simulink model "admire_sim_NDI"  (Simulink 9.1)
settings: Solver=ode4  StartTime=0.0  StopTime=500  FixedStep=dt  RelTol=1e-3  AbsTol=1e-6
InitFcn:
  | INIT_NDI
StartFcn:
  | tic
StopFcn:
  | toctime=toc;
  | fprintf('Actual Time = %g\nSim Time = %g\n',toctime,tout(end))
  | % Make plots
  | %admire_sim_plot
  | figure
  | plot3(yout(:,11),yout(:,10),-yout(:,12),'*-');grid
  | xlabel('East (m)');ylabel('North (m)');zlabel('Alt (m)')
  | view([0 0 1])
  | hold on
  | plot3(Ywpt,Xwpt,0*Xwpt,'r^-','MarkerSize',10)
  | axis equal
  | hold off
values from neighbouring files (symbols this model uses):
  a1 = (180*d2r)/(80^3)    (= 6.13592315154e-06)    [INIT_NDI.m]
  a2 = (24*d2r)/(80^3)    (= 8.18123086872e-07)    [INIT_NDI.m]
  Altcmd_t = [ 0    1   100 200  300  425  450  550  600  700  800  880  980]    [INIT_NDI.m]
  Altcmd_v = [20  20   20   1500 1500 1500 1500 3000 3000 4000 4000 6000 6000]    [INIT_NDI.m]
  bref = 10    [INIT_NDI.m]
  C1 = ((Iy-Iz)*Iz-Ixz^2)/GG    (= -0.958151081688)    [INIT_NDI.m]
  C2 = (Ix-Iy+Iz)*Ixz/GG    (= 0.0484690861804)    [INIT_NDI.m]
  C3 = Iz/GG    (= 4.77597824802e-05)    [INIT_NDI.m]
  C4 = Ixz/GG    (= 1.18217283367e-06)    [INIT_NDI.m]
  C5 = (Iz-Ix)/Iy    (= 0.987654320988)    [INIT_NDI.m]
  C6 = Ixz/Iy    (= 0.0308641975309)    [INIT_NDI.m]
  C7 = 1/Iy    (= 1.23456790123e-05)    [INIT_NDI.m]
  C8 = (Ix*(Ix-Iy)+Ixz^2)/GG    (= -0.592859676085)    [INIT_NDI.m]
  C9 = Ix/GG    (= 9.93025180281e-06)    [INIT_NDI.m]
  CAmethod = 6    [INIT_NDI.m]
  Canard_max = [25 25 25 15 15 15 15 15]*d2r    [INIT_NDI.m]
  Canard_min = [-55 -55 -25 -15 -15 -15 -15 -15]*d2r    [INIT_NDI.m]
  CB = CCV*Bbare    [INIT_NDI.m]
  CC = [C3 0 C4;0 C7 0;C4 0 C9]    [INIT_NDI.m]
  CCV = [CCV zeros(3,22)]    [INIT_NDI.m]
  cref = 5.2    [INIT_NDI.m]
  d2r = pi/180    (= 0.0174532925199)    [INIT_NDI.m]
  dt = 0.01    [INIT_NDI.m]
  DTY_max = 0.002    [INIT_NDI.m]
  DTY_min = -0.002    [INIT_NDI.m]
  DTZ_max = 0.002    [INIT_NDI.m]
  DTZ_min = -0.002    [INIT_NDI.m]
  du = [eye(7,7)*d2r eye(7,7)*(-d2r);zeros(20,14)]    [INIT_NDI.m]
  Elevon_max = [30 30 25 25 25 25 25 25]*d2r    [INIT_NDI.m]
  Elevon_min = [-30 -30 -30 -30 -30 -30 -30 -30]*d2r    [INIT_NDI.m]
  G = [ 0 1 0 ... (first row only)    [INIT_NDI.m]
  kcb = 2.5    [INIT_NDI.m]
  kfb = -0.4    [INIT_NDI.m]
  kib = 0.2    [INIT_NDI.m]
  kpb = 0.8    [INIT_NDI.m]
  LEF_max = [30 30 30 20 20 15 10 10]*d2r    [INIT_NDI.m]
  LEF_min = [-10 -10 -10 -10 -10 -10 -10 -10]*d2r    [INIT_NDI.m]
  LG_max = 1    [INIT_NDI.m]
  LG_min = 0    [INIT_NDI.m]
  LPmethod = 5    [INIT_NDI.m]    (also in LPwrap.m = 0)
  M_vec = [0 0.5 0.8 0.9 0.95 1.4 1.5 2.5]    [INIT_NDI.m]
  mass = 9100    [INIT_NDI.m]
  NumU = 16    [INIT_NDI.m]
  nwpt = 5    [INIT_NDI.m]
  PD_max = 10    [INIT_NDI.m]
  PD_min = -10    [INIT_NDI.m]
  PHIcmd_t = [0 1 1+dt 30 30+dt 60 60+dt 90 90+dt 120 120+dt 150 150+dt 180 180+dt 210 210+dt 240 240+dt 270 270+dt 300 300+dt 330 330+dt]    [INIT_NDI.m]
  PHIcmd_v = [0 0 15   15 -15   -15 0    0   30   30  -30    -30 0      0   45     45   0     0    -45   -45   0     0   -60   -60 0]    [INIT_NDI.m]
  Pmode = 3    [INIT_NDI.m]
  r2d = 180/pi    (= 57.2957795131)    [INIT_NDI.m]
  Rmode = 3    [INIT_NDI.m]
  Rudder_max = [30 30 25 20 15 15 15 10]*d2r    [INIT_NDI.m]
  Rudder_min = [-30 -30 -25 -20 -15 -15 -15 -10]*d2r    [INIT_NDI.m]
  Sref = 45    [INIT_NDI.m]
  TSS_max = 1    [INIT_NDI.m]
  TSS_min = 0    [INIT_NDI.m]
  UD_max = 10    [INIT_NDI.m]
  UD_min = -10    [INIT_NDI.m]
  Upref = [0 0 0 0 0 0 0 0 0 0 0 0 0 0 0 0]'    [INIT_NDI.m]
  Upref_split = [[0 0 30 -30 -30 30 0]*d2r*.4 0 0 0 0 0 0 0 0 0]'    [INIT_NDI.m]
  Urlim = [50*d2r ... (first row only)    [INIT_NDI.m]
  UseRL = 0    [INIT_NDI.m]
  Vcmd_t = [  0    1   100  200  300  425  450  550  600  700  800  880  980]    [INIT_NDI.m]
  Vcmd_v = Mcmd_v.*a    [INIT_NDI.m]
  VD_max = 10    [INIT_NDI.m]
  VD_min = -10    [INIT_NDI.m]
  WD_max = 10    [INIT_NDI.m]
  WD_min = -10    [INIT_NDI.m]
  Wp = W'*W    [INIT_NDI.m]
  Wpts = [0 1 2 3 4]    [INIT_NDI.m]
  x0 = [ max(eyp,zeros(n,1));max(-eyp,zeros(n,1));zeros(2*m,1)]    [LPwrap.m]
  Xwpt = [0 4000 4000 0 0]*8    [INIT_NDI.m]
  Ywpt = [0 0 4000 4000 0]*8    [INIT_NDI.m]
undefined symbols (not defined in the file or in its folder): Abare, Bbare, CGIwrap, dalpha_err, dalt_err, DAwrap, dbeta_err, ddc_bw, ddc_rate, ddei_bw, ddei_rate, ddey_bw, ddey_rate, ddle_bw, ddle_rate, ddr_bw, ddr_rate, DiscIntNeverNeededParam, dVt_err, LPwrap, rlimit_c, rlimit_ie, rlimit_le, rlimit_oe, rlimit_r, u0fcs, u0new, VJAwrap, x0bare, y0bare
libraries: simulink_extras x19, simulink x12
(part 3 of 4)

== system admire_sim_NDI/NDI_CLAW/DynamicInversionControl/REG/PitchReg/QCMD_1 ==
  CMD : Inport
  INPUT : Inport  Port=2
  Action Port : ActionPort  ActionType=then
  1-D Lookup Table : Lookup_n-D  NumberOfTableDimensions=1  BreakpointsForDimension1=[0.4 0.6 0.8]  Table=[30 40 50]  ExtrapMethod=Clip  UseLastTableValue=on  RndMeth=Simplest  InputSameDT=on
  Bus Selector1 : BusSelector  OutputSignals=PSTICK
  Bus Selector2 : BusSelector  OutputSignals=Mach
  Bus Selector4 : BusSelector  OutputSignals=Qb_rps
  Bus Selector5 : BusSelector  OutputSignals=Reset
  Discrete-Time Integrator1 : DiscreteIntegrator  IntegratorMethod=Integration: Trapezoidal  ExternalReset=level  SampleTime=dt  ICPrevOutput=DiscIntNeverNeededParam  ICPrevScaledInput=DiscIntNeverNeededParam
  Gain2 : Gain  Gain=6
  Gain3 : Gain  Gain=5
  Gain4 : Gain  Gain=d2r
  Gain5 : Gain  Gain=-1
  Gain6 : Gain  Gain=80
  Product : Product  RndMeth=Zero
  QCMD_Gradient : Lookup_n-D  NumberOfTableDimensions=1  BreakpointsForDimension1=[-80:80]  Table=a2*([-80:80].^3)  ExtrapMethod=Clip  UseLastTableValue=on  RndMeth=Simplest  InputSameDT=on
  Sum : Sum  Inputs=+++
  Sum2 : Sum  Inputs=|+-
  MCVdt : Outport
  wires:
  CMD/1 -> Bus Selector1/1, Bus Selector5/1
  QCMD_Gradient/1 -> Sum2/1, Gain5/1  "Qcmd"
  Sum2/1 -> Gain2/1, Gain3/1
  Sum/1 -> MCVdt/1  "QDT_des"
  INPUT/1 -> Bus Selector2/1, Bus Selector4/1
  Bus Selector2/1 -> 1-D Lookup Table/1  "<Mach>"
  1-D Lookup Table/1 -> Product/2
  Bus Selector1/1 -> Gain6/1, Product/1  "<PSTICK>"
  Product/1 -> Gain4/1
  Bus Selector5/1 -> Discrete-Time Integrator1/2  "<Reset>"
  Discrete-Time Integrator1/1 -> Sum/2
  Gain2/1 -> Sum/3
  Gain3/1 -> Discrete-Time Integrator1/1
  Gain5/1 -> Sum/1
  Gain6/1 -> QCMD_Gradient/1
  Bus Selector4/1 -> Sum2/2  "<Qb_rps>"

== system admire_sim_NDI/NDI_CLAW/DynamicInversionControl/REG/RollReg/PHIcmd_2 ==
  CMD : Inport
  INPUT : Inport  Port=2
  Action Port : ActionPort  ActionType=elseif
  Bus Selector2 : BusSelector  OutputSignals=PHIcmd_rad
  Bus Selector3 : BusSelector  OutputSignals=PHI_rad
  Bus Selector5 : BusSelector  OutputSignals=Reset
  Constant : Constant  Value=100*d2r
  Discrete-Time Integrator1 : DiscreteIntegrator  IntegratorMethod=Integration: Trapezoidal  ExternalReset=level  SampleTime=dt  ICPrevOutput=DiscIntNeverNeededParam  ICPrevScaledInput=DiscIntNeverNeededParam
  Gain1 : Gain  Gain=5
  Gain3 : Gain  Gain=1.6
  Gain7 : Gain  Gain=-0.8
  Gain8 : Gain  Gain=.8
  Get_LCV : Subsystem
  Sum1 : Sum  Inputs=|+-
  Sum2 : Sum  Inputs=|+-
  Sum3 : Sum  Inputs=++|
  Sum4 : Sum  Inputs=++|
  VariableLimiter : Subsystem
  LCVdt : Outport
  wires:
  CMD/1 -> Bus Selector5/1, Bus Selector2/1
  Sum1/1 -> Gain8/1, Gain3/1
  Bus Selector3/1 -> Sum1/2  "<PHI_rad>"
  Sum2/1 -> Gain1/1
  Gain1/1 -> LCVdt/1  "Pdt_des"
  VariableLimiter/1(Out) -> Sum2/1  "Pcmd_lim"
  Constant/1 -> VariableLimiter/2(Limit)
  Get_LCV/1(LCV) -> Sum2/2
  INPUT/1 -> Get_LCV/1(Input), Bus Selector3/1
  Bus Selector5/1 -> Discrete-Time Integrator1/2  "<Reset>"
  Gain3/1 -> Sum4/2  "Pcmd"
  Sum4/1 -> VariableLimiter/1(Input)
  Gain8/1 -> Discrete-Time Integrator1/1
  Discrete-Time Integrator1/1 -> Sum3/2
  Sum3/1 -> Sum4/1
  Gain7/1 -> Sum3/1
  Bus Selector2/1 -> Sum1/1, Gain7/1  "<PHIcmd_rad>"

== system admire_sim_NDI/NDI_CLAW/DynamicInversionControl/REG/RollReg/Pcmd_1 ==
  CMD : Inport
  INPUT : Inport  Port=2
  Action Port : ActionPort  ActionType=then
  1-D Lookup Table : Lookup_n-D  NumberOfTableDimensions=1  BreakpointsForDimension1=[0.4 0.6 0.8]  Table=[50 100 180]  ExtrapMethod=Clip  UseLastTableValue=on  RndMeth=Simplest  InputSameDT=on
  Bus Selector2 : BusSelector  OutputSignals=RSTICK
  Bus Selector3 : BusSelector  OutputSignals=Mach
  Constant : Constant  Value=100*d2r
  Gain1 : Gain  Gain=2
  Gain2 : Gain  Gain=d2r
  Gain3 : Gain  Gain=80
  Get_LCV : Subsystem
  PCMD_Gradient : Lookup_n-D  NumberOfTableDimensions=1  BreakpointsForDimension1=[-80:80]  Table=a1*([-80:80].^3)  ExtrapMethod=Clip  UseLastTableValue=on  RndMeth=Simplest  InputSameDT=on
  Product : Product  RndMeth=Zero
  Sum2 : Sum  Inputs=|+-
  Terminator : Terminator
  VariableLimiter : Subsystem
  LCVdt : Outport
  wires:
  Get_LCV/1(LCV) -> Sum2/2
  PCMD_Gradient/1 -> Sum2/1  "Pcmd_lim"
  Gain1/1 -> LCVdt/1  "Pdt_des"
  Sum2/1 -> Gain1/1
  Product/1 -> Gain2/1  "Pcmd_dps"
  Bus Selector2/1 -> Product/1, Gain3/1  "<RSTICK>"
  CMD/1 -> Bus Selector2/1
  Gain2/1 -> VariableLimiter/1(Input)  "Pcmd_rps"
  INPUT/1 -> Get_LCV/1(Input), Bus Selector3/1
  Bus Selector3/1 -> 1-D Lookup Table/1  "<Mach>"
  1-D Lookup Table/1 -> Product/2
  Constant/1 -> VariableLimiter/2(Limit)
  Gain3/1 -> PCMD_Gradient/1
  VariableLimiter/1(Out) -> Terminator/1  "Pcmd_lim"

== system admire_sim_NDI/NDI_CLAW/DynamicInversionControl/REG/RollReg/XTKcmd_3 ==
  CMD : Inport
  INPUT : Inport  Port=2
  Action Port : ActionPort  ActionType=else
  Bus Selector3 : BusSelector  OutputSignals=PHI_rad
  Constant : Constant  Value=100*d2r
  Gain1 : Gain  Gain=3
  Gain3 : Gain  Gain=.75
  GetPHIcmd : Subsystem
  Get_LCV : Subsystem
  Sum1 : Sum  Inputs=|+-
  Sum2 : Sum  Inputs=|+-
  VariableLimiter : Subsystem
  LCVdt : Outport
  wires:
  Get_LCV/1(LCV) -> Sum2/2
  Constant/1 -> VariableLimiter/2(Limit)
  VariableLimiter/1(Out) -> Sum2/1  "Pcmd_lim"
  Gain1/1 -> LCVdt/1  "Pdt_des"
  Sum2/1 -> Gain1/1
  Bus Selector3/1 -> Sum1/2  "<PHI_rad>"
  Gain3/1 -> VariableLimiter/1(Input)  "Pcmd"
  Sum1/1 -> Gain3/1
  GetPHIcmd/1(PHIcmd) -> Sum1/1
  CMD/1 -> GetPHIcmd/1(CMD)
  INPUT/1 -> Get_LCV/1(Input), Bus Selector3/1, GetPHIcmd/2(INPUT)

== system admire_sim_NDI/NDI_CLAW/DynamicInversionControl/REG/YawReg/Get_NCV ==
  Input : Inport
  Bus Selector4 : BusSelector  OutputSignals=Rb_rps,ALPHA_rad,Pb_rps,VT_mps,PHI_rad,THETA_rad
  Constant : Constant
  Gain : Gain  Gain=9.81
  MinMax : MinMax  Function=max  Inputs=2
  Product : Product  RndMeth=Zero
  Product1 : Product  RndMeth=Zero
  Product2 : Product  Inputs=/**  RndMeth=Zero
  Sum4 : Sum  Inputs=|+-
  Sum5 : Sum  Inputs=|+-
  Trigonometric Function : Trigonometry
  Trigonometric Function1 : Trigonometry  Operator=cos
  Trigonometric Function2 : Trigonometry
  Trigonometric Function3 : Trigonometry  Operator=cos
  NCV : Outport
  wires:
  Bus Selector4/2 -> Trigonometric Function/1, Trigonometric Function1/1  "<ALPHA_rad>"
  Trigonometric Function1/1 -> Product/2
  Trigonometric Function/1 -> Product1/1
  Product/1 -> Sum4/1
  Product1/1 -> Sum4/2
  Constant/1 -> MinMax/2
  Bus Selector4/4 -> MinMax/1  "<VT_mps>"
  Bus Selector4/5 -> Trigonometric Function2/1  "<PHI_rad>"
  Bus Selector4/6 -> Trigonometric Function3/1  "<THETA_rad>"
  MinMax/1 -> Product2/1
  Trigonometric Function2/1 -> Product2/2
  Trigonometric Function3/1 -> Product2/3
  Product2/1 -> Gain/1
  Sum4/1 -> Sum5/1
  Gain/1 -> Sum5/2
  Input/1 -> Bus Selector4/1
  Bus Selector4/1 -> Product/1  "<Rb_rps>"
  Bus Selector4/3 -> Product1/2  "<Pb_rps>"
  Sum5/1 -> NCV/1

== system admire_sim_NDI/NDI_CLAW/MissionManager/WaypointNavigation/ChangeWptNumber/GetTurnDist ==
  INPUT : Inport
  WNz : Inport  Port=2
  Bus Selector2 : BusSelector  OutputSignals=VT_mps  OutputAsBus=on
  GetHalfAngle : Subsystem
  GetPHILimit : Subsystem
  GetRadius : Subsystem
  Product : Product  RndMeth=Zero
  Product4 : Product  Inputs=**/  RndMeth=Zero
  Trigonometric Function1 : Trigonometry  Operator=cos
  Trigonometric Function2 : Trigonometry
  V2 : Outport
  TurnDist_m : Outport  Port=2
  PHImax_rad : Outport  Port=3
  wires:
  Bus Selector2/1 -> Product/1, Product/2
  Product/1 -> V2/1, GetRadius/1(V2), GetPHILimit/1(V2)
  GetPHILimit/1(PHImax_rad) -> GetRadius/2(PHImax_rad), PHImax_rad/1
  INPUT/1 -> Bus Selector2/1
  WNz/1 -> GetHalfAngle/1(WNz)
  GetHalfAngle/1(Out1) -> Trigonometric Function1/1, Trigonometric Function2/1
  GetRadius/1(R_m) -> Product4/1
  Trigonometric Function1/1 -> Product4/2
  Trigonometric Function2/1 -> Product4/3
  Product4/1 -> TurnDist_m/1  "TurnDist_m"

== system admire_sim_NDI/NDI_CLAW/DynamicInversionControl/AERO_OBM/NonLinearOBM/Get_B_Aero/Dimensions ==
  note: Generate a matrix which will multiply
      | the moment coefficients to turn them
      | into properly dimensioned moments
  In1 : Inport
  Gain1 : Gain  Gain=-1
  Gain2 : Gain  Gain=0.5
  Gain3 : Gain  Gain=bref
  Gain4 : Gain  Gain=bref
  Gain5 : Gain  Gain=cref
  Gain6 : Gain  Gain=Sref
  Gain7 : Gain  Gain=[1 1 1]  Multiplication=Matrix(u*K)
  Gain8 : Gain  Gain=eye(3,3)
  GetDensity : Subsystem
  Mux1 : Mux  Inputs=3
  Product : Product  RndMeth=Zero
  Product1 : Product  RndMeth=Zero
  Selector4 : Selector  InputPortWidth=27  IndexOptions=Index vector (dialog)  Indices=[19]  OutputSizes=1
  Selector5 : Selector  InputPortWidth=27  IndexOptions=Index vector (dialog)  Indices=[13]  OutputSizes=1
  Out1 : Outport
  wires:
  Selector4/1 -> Gain1/1
  Gain1/1 -> GetDensity/1(Alt_m)  "Alt_m"
  Selector5/1 -> Product/1, Product/2
  Product/1 -> Gain2/1
  GetDensity/1(rho_kpm3) -> Product1/1
  Gain2/1 -> Product1/2  "V*V*0.5"
  Gain5/1 -> Mux1/2
  Gain3/1 -> Mux1/1
  Gain4/1 -> Mux1/3
  Product1/1 -> Gain3/1, Gain5/1, Gain4/1  "dynamic pressure"
  Mux1/1 -> Gain6/1
  In1/1 -> Selector4/1, Selector5/1
  Gain6/1 -> Gain7/1
  Gain7/1 -> Gain8/1
  Gain8/1 -> Out1/1

== system admire_sim_NDI/NDI_CLAW/DynamicInversionControl/AERO_OBM/NonLinearOBM/Get_B_Aero/Get_CVdt ==
  Dim : Inport
  Sensors : Inport  Port=2
  uz : Inport  Port=3
  DueToEffectors : Subsystem
  Sum : Sum  Inputs=|+-
  TotalAccels : Subsystem
  CVdt : Outport
  wires:
  DueToEffectors/1(Out1) -> Sum/2  "B*u-B*u_nom"
  Sum/1 -> CVdt/1
  uz/1 -> DueToEffectors/3(uz)
  Dim/1 -> DueToEffectors/2(Dim), TotalAccels/1(Dim)
  Sensors/1 -> DueToEffectors/1(Sensors), TotalAccels/2(Sensors)
  TotalAccels/1(CVdt) -> Sum/1  "f(x,u)"

== system admire_sim_NDI/NDI_CLAW/DynamicInversionControl/AERO_OBM/NonLinearOBM/Get_B_Aero/OneColPerFrame ==
  In1 : Inport
  In2 : Inport  Port=2
  Bz : Inport  Port=3
  Assignment : Assignment  NumberOfDimensions=2  IndexOptions=Index vector (dialog),Index vector (port)  Indices=[1 2 3],1  OutputSizes=1,1
  Merge : Merge  Inputs=7
  Signal Specification : SignalSpecification  Dimensions=[3 1]
  Switch Case : SwitchCase  CaseConditions={7,6,5,4,3,2,1}  ShowDefaultCase=off  SampleTime=0
  u1 : Subsystem
  u2 : Subsystem
  u3 : Subsystem
  u4 : Subsystem
  u5 : Subsystem
  u6 : Subsystem
  u7 : Subsystem
  Out1 : Outport
  wires:
  In1/1 -> u1/1(In1), u2/1(In1), u3/1(In1), u4/1(In1), u5/1(In1), u7/1(In1), u6/1(In1)
  u1/1(Out1) -> Merge/1
  u2/1(Out1) -> Merge/2
  u3/1(Out1) -> Merge/3
  u4/1(Out1) -> Merge/4
  u5/1(Out1) -> Merge/5
  u6/1(Out1) -> Merge/6
  u7/1(Out1) -> Merge/7
  Switch Case/1 -> u7/Action
  Switch Case/2 -> u6/Action
  Switch Case/3 -> u5/Action
  Switch Case/4 -> u4/Action
  Switch Case/5 -> u3/Action
  Switch Case/6 -> u2/Action
  Switch Case/7 -> u1/Action
  In2/1 -> Assignment/3, Switch Case/1
  Bz/1 -> Assignment/1
  Assignment/1 -> Out1/1
  Merge/1 -> Signal Specification/1
  Signal Specification/1 -> Assignment/2

== system admire_sim_NDI/NDI_CLAW/DynamicInversionControl/ControlAllocation/GetU/MakeSquare_0/Subsystem ==
  In1 : Inport
  Bus Selector1 : BusSelector  OutputSignals=CB
  Bus Selector3 : BusSelector  OutputSignals=INDX
  Constant : Constant  Value=G
  Math Function2 : Math  Operator=transpose  SaturateOnIntegerOverflow=on
  Matrix Concatenate : Concatenate  NumInputs=3  Mode=Multidimensional array
  Product : Product
  Product1 : Product  Multiplication=Matrix(*)
  Signal Specification1 : SignalSpecification  Dimensions=[1 NumU]
  Gmod : Outport
  CBGmod : Outport  Port=2
  wires:
  Math Function2/1 -> Product/2
  Bus Selector3/1 -> Signal Specification1/1  "<INDX>"
  Signal Specification1/1 -> Matrix Concatenate/1, Matrix Concatenate/2, Matrix Concatenate/3
  Product/1 -> Product1/2, Gmod/1
  Matrix Concatenate/1 -> Math Function2/1
  Constant/1 -> Product/1
  Bus Selector1/1 -> Product1/1  "<CB>"
  In1/1 -> Bus Selector1/1, Bus Selector3/1
  Product1/1 -> CBGmod/1

== system admire_sim_NDI/NDI_CLAW/DynamicInversionControl/ControlAllocation/GetU/WeightedPseudo Clipped_1/GetP ==
  CB : Inport
  WpT : Inport  Port=2
  CBT : Inport  Port=3
  Product : Product  Inputs=/*  Multiplication=Matrix(*)  RndMeth=Zero
  Product1 : Product  Inputs=**  Multiplication=Matrix(*)  RndMeth=Zero
  Product2 : Product  Inputs=*/  Multiplication=Matrix(*)  RndMeth=Zero
  P : Outport
  wires:
  CBT/1 -> Product/2
  Product2/1 -> P/1  "P"
  WpT/1 -> Product/1
  CB/1 -> Product1/1
  Product1/1 -> Product2/2
  Product/1 -> Product2/1, Product1/2

== system admire_sim_NDI/NDI_CLAW/DynamicInversionControl/ControlAllocation/GetU/WeightedPseudo Clipped_1/SelectActive ==
  In1 : Inport
  Bus Selector2 : BusSelector  OutputSignals=CB
  Bus Selector3 : BusSelector  OutputSignals=INDX
  Matrix Concatenate : Concatenate  NumInputs=3  Mode=Multidimensional array
  Product : Product
  Signal Specification1 : SignalSpecification  Dimensions=[1 NumU]
  Out1 : Outport
  wires:
  Matrix Concatenate/1 -> Product/1
  Product/1 -> Out1/1
  Bus Selector3/1 -> Signal Specification1/1  "<INDX>"
  Bus Selector2/1 -> Product/2  "<CB>"
  In1/1 -> Bus Selector3/1, Bus Selector2/1
  Signal Specification1/1 -> Matrix Concatenate/3, Matrix Concatenate/2, Matrix Concatenate/1

== system admire_sim_NDI/NDI_CLAW/DynamicInversionControl/ControlAllocation/GetU/WeightedPseudo Scaled_2/Blocks ==
  CB : Inport
  CVdt_des : Inport  Port=2
  Umin : Inport  Port=3
  Umax : Inport  Port=4
  Wp : Inport  Port=5
  CheckSaturation : Subsystem
  GetP : Subsystem
  If : If  IfExpression=u1 < 1
  Math Function : Math  Operator=transpose  SaturateOnIntegerOverflow=on
  Math Function1 : Math  Operator=transpose  SaturateOnIntegerOverflow=on
  Merge : Merge
  None_Saturated : Subsystem  TreatAsAtomicUnit=on
  Product3 : Product  Inputs=**  Multiplication=Matrix(*)  RndMeth=Zero
  Some_Saturated : Subsystem  TreatAsAtomicUnit=on
  Out1 : Outport
  wires:
  Merge/1 -> Out1/1
  Umin/1 -> Some_Saturated/2(umin), CheckSaturation/2(Umin)
  Umax/1 -> Some_Saturated/1(umax), CheckSaturation/3(Umax)
  None_Saturated/1(Out1) -> Merge/2
  Some_Saturated/1(Out1) -> Merge/1
  If/1 -> None_Saturated/Action
  If/2 -> Some_Saturated/Action
  CheckSaturation/1(Out1) -> If/1
  Product3/1 -> CheckSaturation/1(In1), Some_Saturated/3(u), None_Saturated/1(In1)  "u"
  CVdt_des/1 -> Product3/2
  GetP/1(P) -> Product3/1
  Math Function1/1 -> GetP/3(CBT)
  Math Function/1 -> GetP/2(WpT)
  Wp/1 -> Math Function/1
  CB/1 -> GetP/1(CB), Math Function1/1

== system admire_sim_NDI/NDI_CLAW/DynamicInversionControl/ControlAllocation/GetU/WeightedPseudo Scaled_2/SelectActive ==
  In1 : Inport
  Bus Selector2 : BusSelector  OutputSignals=CB
  Bus Selector3 : BusSelector  OutputSignals=INDX
  Matrix Concatenate : Concatenate  NumInputs=3  Mode=Multidimensional array
  Product : Product
  Signal Specification1 : SignalSpecification  Dimensions=[1 NumU]
  Out1 : Outport
  wires:
  Matrix Concatenate/1 -> Product/1
  Product/1 -> Out1/1
  Bus Selector3/1 -> Signal Specification1/1  "<INDX>"
  Bus Selector2/1 -> Product/2  "<CB>"
  In1/1 -> Bus Selector3/1, Bus Selector2/1
  Signal Specification1/1 -> Matrix Concatenate/3, Matrix Concatenate/2, Matrix Concatenate/1

== system admire_sim_NDI/NDI_CLAW/DynamicInversionControl/ControlAllocation/PostProcess/DriveToPreferred/Get_UPerp ==
  In1 : Inport
  In2 : Inport  Port=2
  Bus Selector3 : BusSelector  OutputSignals=CB,INDX
  MATLAB Fcn : MATLABFcn  MATLABFcn=getUperp  Output1D=off
  Math Function1 : Math  Operator=transpose  SaturateOnIntegerOverflow=on
  Math Function3 : Math  Operator=transpose  SaturateOnIntegerOverflow=on
  Matrix Concatenate : Concatenate  NumInputs=3  Mode=Multidimensional array
  Signal Specification1 : SignalSpecification  Dimensions=[NumU 1]
  Signal Specification3 : SignalSpecification  Dimensions=[NumU 1]
  Out1 : Outport
  wires:
  Signal Specification3/1 -> Math Function3/1
  Matrix Concatenate/1 -> MATLAB Fcn/1
  In1/1 -> Bus Selector3/1
  Bus Selector3/2 -> Signal Specification3/1  "<INDX>"
  MATLAB Fcn/1 -> Out1/1
  Bus Selector3/1 -> Matrix Concatenate/1  "<CB>"
  In2/1 -> Signal Specification1/1
  Signal Specification1/1 -> Math Function1/1
  Math Function1/1 -> Matrix Concatenate/2
  Math Function3/1 -> Matrix Concatenate/3

== system admire_sim_NDI/NDI_CLAW/DynamicInversionControl/ControlAllocation/PostProcess/DriveToPreferred/LimitScale ==
  note: Deal with the situation where K_opt*u_perp is already the optimal solution, at this time the gain is greater than 1
  Vector : Inport
  MinValues : Inport  Port=2
  MaxValues : Inport  Port=3
  PrePro : Inport  Port=4
  Abs1 : Abs
  "Calculate the gain factor to the lower limit " : Subsystem
  "Calculate the gain factor to the upper limit " : Subsystem
  Compare To Zero : simulink/Logic and Bit Operations/Compare To Zero  relop=<  OutDataTypeStr=uint8
  Compare To Zero1 : simulink/Logic and Bit Operations/Compare To Zero  relop=>=  OutDataTypeStr=uint8
  Constant : Constant
  Data Type Conversion1 : DataTypeConversion  OutDataTypeStr=double
  Data Type Conversion2 : DataTypeConversion  OutDataTypeStr=double
  DivideByZeroProtection : Subsystem
  MinMax : MinMax
  Mux : Mux  Inputs=2
  Product : Product  RndMeth=Zero
  Product1 : Product  RndMeth=Zero
  Sign : Signum
  Sum : Sum  Inputs=|++
  Scale : Outport
  wires:
  Abs1/1 -> MinMax/1
  MinMax/1 -> Scale/1
  Vector/1 -> DivideByZeroProtection/1(In1)
  DivideByZeroProtection/1(Out1) -> "Calculate the gain factor to the lower limit "/1(oou), Sign/1, "Calculate the gain factor to the upper limit "/3(oou)
  MaxValues/1 -> "Calculate the gain factor to the lower limit "/2(MaxValues)
  Mux/1 -> Abs1/1
  Constant/1 -> Mux/2
  PrePro/1 -> "Calculate the gain factor to the lower limit "/3(PrePro), "Calculate the gain factor to the upper limit "/1(PrePro)
  MinValues/1 -> "Calculate the gain factor to the upper limit "/2(MinValues)
  Sign/1 -> Compare To Zero1/1, Compare To Zero/1
  Compare To Zero/1 -> Data Type Conversion1/1
  Data Type Conversion1/1 -> Product/2
  "Calculate the gain factor to the upper limit "/1(Out1) -> Product/1
  Product/1 -> Sum/1
  Compare To Zero1/1 -> Data Type Conversion2/1
  Data Type Conversion2/1 -> Product1/1
  "Calculate the gain factor to the lower limit "/1(Out1) -> Product1/2
  Product1/1 -> Sum/2
  Sum/1 -> Mux/1

== system admire_sim_NDI/NDI_CLAW/DynamicInversionControl/ControlAllocation/PostProcess/DriveToPreferred/displaced origin ==
  u : Inport
  PrePro : Inport  Port=2
  Bus Selector1 : BusSelector  OutputSignals=Umax
  Bus Selector3 : BusSelector  OutputSignals=Umin
  Sum1 : Sum  Inputs=-+|
  Sum4 : Sum  Inputs=|+-
  MinV : Outport
  MaxV : Outport  Port=2
  wires:
  Bus Selector3/1 -> Sum4/1  "<Umin>"
  PrePro/1 -> Bus Selector3/1, Bus Selector1/1
  Sum4/1 -> MinV/1
  u/1 -> Sum4/2, Sum1/1
  Bus Selector1/1 -> Sum1/2  "<Umax>"
  Sum1/1 -> MaxV/1

== system admire_sim_NDI/NDI_CLAW/DynamicInversionControl/ControlAllocation/PreProcess/GetLimits/PositionAndRateLimited ==
  In1 : Inport
  Action Port : ActionPort  ActionType=else
  Bus Selector1 : BusSelector  OutputSignals=Umax
  Bus Selector2 : BusSelector  OutputSignals=Umin
  Bus Selector3 : BusSelector  OutputSignals=Unom
  Bus Selector4 : BusSelector  OutputSignals=Unom
  Constant : Constant  Value=-Urlim*dt
  Constant1 : Constant  Value=Urlim*dt
  Gain : Gain
  Gain1 : Gain
  MinMax : MinMax  Function=max  Inputs=2
  MinMax1 : MinMax  Inputs=2
  Sum : Sum  Inputs=|-+
  Sum1 : Sum  Inputs=|+-
  Umin : Outport
  Umax : Outport  Port=2
  wires:
  Bus Selector2/1 -> Sum/2  "<Umin>"
  Bus Selector1/1 -> Sum1/1  "<Umax>"
  In1/1 -> Bus Selector2/1, Bus Selector3/1, Bus Selector1/1, Bus Selector4/1
  Gain/1 -> Umin/1
  Gain1/1 -> Umax/1
  Bus Selector3/1 -> Sum/1  "<Unom>"
  Constant/1 -> MinMax/1
  MinMax/1 -> Gain/1
  Sum/1 -> MinMax/2
  Bus Selector4/1 -> Sum1/2  "<Unom>"
  Sum1/1 -> MinMax1/1
  Constant1/1 -> MinMax1/2
  MinMax1/1 -> Gain1/1

== system admire_sim_NDI/NDI_CLAW/DynamicInversionControl/ControlAllocation/PreProcess/GetLimits/PositionLimited ==
  In1 : Inport
  Action Port : ActionPort  ActionType=then
  Bus Selector3 : BusSelector  OutputSignals=Umax
  Bus Selector4 : BusSelector  OutputSignals=Umin
  Bus Selector5 : BusSelector  OutputSignals=Unom
  Bus Selector6 : BusSelector  OutputSignals=Unom
  Gain : Gain
  Gain1 : Gain
  Sum : Sum  Inputs=|-+
  Sum1 : Sum  Inputs=|+-
  Umax : Outport
  Umin : Outport  Port=2
  wires:
  Sum/1 -> Gain/1
  Sum1/1 -> Gain1/1
  Gain/1 -> Umin/1
  Gain1/1 -> Umax/1
  Bus Selector4/1 -> Sum/2  "<Umin>"
  Bus Selector3/1 -> Sum1/1  "<Umax>"
  Bus Selector5/1 -> Sum/1  "<Unom>"
  Bus Selector6/1 -> Sum1/2  "<Unom>"
  In1/1 -> Bus Selector5/1, Bus Selector4/1, Bus Selector3/1, Bus Selector6/1

== system admire_sim_NDI/NDI_CLAW/DynamicInversionControl/REG/PitchReg/ALTCMD_3/Discrete TFz 1st Order1 ==
  IN : Inport
  Sum : Sum  Inputs=|+-
  Sum1 : Sum  Inputs=++|
  Unit Delay : UnitDelay  InitialCondition=UnitDelay  SampleTime=-1
  dz2 : Gain  Gain=denz(2)  OutDataTypeStr=double
  nz1 : Gain  Gain=numz(1)
  nz2 : Gain  Gain=numz(2)
  oodz1 : Gain  Gain=1/denz(1)
  OUT : Outport
  wires:
  oodz1/1 -> OUT/1, dz2/1
  Sum1/1 -> oodz1/1
  nz1/1 -> Sum1/1
  nz2/1 -> Sum/1
  IN/1 -> nz2/1, nz1/1
  Sum/1 -> Unit Delay/1
  Unit Delay/1 -> Sum1/2
  dz2/1 -> Sum/2

== system admire_sim_NDI/NDI_CLAW/DynamicInversionControl/REG/PitchReg/ALTCMD_3/GetGammas ==
  ANGLES : Inport
  Bus Selector1 : BusSelector  OutputSignals=ALPHA_rad,BETA_rad,THETA_rad
  Bus Selector2 : BusSelector  OutputSignals=PHI_rad,BETA_rad
  Bus Selector3 : BusSelector  OutputSignals=PHI_rad,ALPHA_rad,BETA_rad
  Bus Selector4 : BusSelector  OutputSignals=THETA_rad
  Product : Product  Inputs=3  RndMeth=Zero
  Product1 : Product  RndMeth=Zero
  Product2 : Product  Inputs=3  RndMeth=Zero
  Product3 : Product  RndMeth=Zero
  Sum : Sum  Inputs=|+-
  Sum1 : Sum  Inputs=|++
  Trigonometric Function{1,5..7,9} (5 alike) : Trigonometry  Operator=cos
  Trigonometric Function10 : Trigonometry  Operator=asin
  Trigonometric Function{2..4,8} (4 alike) : Trigonometry
  GAMMA_rad : Outport
  wires:
  Trigonometric Function10/1 -> GAMMA_rad/1  "GAMMA_rad"
  Trigonometric Function7/1 -> Product3/1
  Product3/1 -> Sum/2
  Product/1 -> Sum/1
  Sum1/1 -> Product3/2
  Bus Selector4/1 -> Trigonometric Function7/1  "<THETA_rad>"
  Product2/1 -> Sum1/2
  Product1/1 -> Sum1/1
  Bus Selector3/3 -> Trigonometric Function5/1  "<BETA_rad>"
  Bus Selector3/1 -> Trigonometric Function6/1  "<PHI_rad>"
  Trigonometric Function5/1 -> Product2/3
  Trigonometric Function4/1 -> Product2/2
  Trigonometric Function6/1 -> Product2/1
  Bus Selector3/2 -> Trigonometric Function4/1  "<ALPHA_rad>"
  Trigonometric Function3/1 -> Product1/2
  Trigonometric Function2/1 -> Product1/1
  Bus Selector2/2 -> Trigonometric Function3/1  "<BETA_rad>"
  Bus Selector2/1 -> Trigonometric Function2/1  "<PHI_rad>"
  Trigonometric Function8/1 -> Product/3
  Trigonometric Function1/1 -> Product/2
  Trigonometric Function9/1 -> Product/1
  Bus Selector1/3 -> Trigonometric Function8/1  "<THETA_rad>"
  Bus Selector1/2 -> Trigonometric Function1/1  "<BETA_rad>"
  Bus Selector1/1 -> Trigonometric Function9/1  "<ALPHA_rad>"
  ANGLES/1 -> Bus Selector4/1, Bus Selector1/1, Bus Selector3/1, Bus Selector2/1
  Sum/1 -> Trigonometric Function10/1

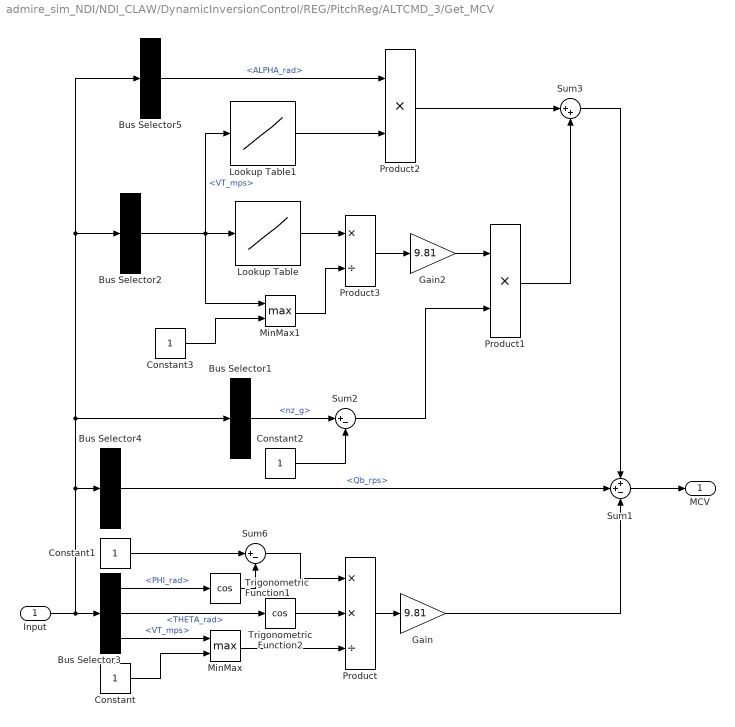
== system admire_sim_NDI/NDI_CLAW/DynamicInversionControl/REG/PitchReg/ALTCMD_3/Get_MCV ==
  Input : Inport
  Bus Selector1 : BusSelector  OutputSignals=nz_g
  Bus Selector2 : BusSelector  OutputSignals=VT_mps
  Bus Selector3 : BusSelector  OutputSignals=PHI_rad,THETA_rad,VT_mps
  Bus Selector4 : BusSelector  OutputSignals=Qb_rps
  Bus Selector5 : BusSelector  OutputSignals=ALPHA_rad
  Constant{,1..3} (4 alike) : Constant
  Gain : Gain  Gain=9.81
  Gain2 : Gain  Gain=9.81
  Lookup Table : Lookup  InputValues=[0 140 150 200 250]  Table=[0 0 1 1 1]*0.  LookUpMeth=Interpolation-Use End Values
  Lookup Table1 : Lookup  InputValues=[0 140 150 200 250]  Table=[0 0 1 1 1]*0.  LookUpMeth=Interpolation-Use End Values
  MinMax : MinMax  Function=max  Inputs=2
  MinMax1 : MinMax  Function=max  Inputs=2
  Product : Product  Inputs=**/  RndMeth=Zero
  Product1 : Product  Inputs=**  RndMeth=Zero
  Product2 : Product  Inputs=**  RndMeth=Zero
  Product3 : Product  Inputs=*/  RndMeth=Zero
  Sum1 : Sum  Inputs=++-
  Sum2 : Sum  Inputs=|+-
  Sum3 : Sum  Inputs=|++
  Sum6 : Sum  Inputs=|+-
  Trigonometric Function1 : Trigonometry  Operator=cos
  Trigonometric Function2 : Trigonometry  Operator=cos
  MCV : Outport
  wires:
  Bus Selector3/3 -> MinMax/1  "<VT_mps>"
  Constant/1 -> MinMax/2
  Bus Selector3/1 -> Trigonometric Function1/1  "<PHI_rad>"
  Bus Selector3/2 -> Trigonometric Function2/1  "<THETA_rad>"
  Product/1 -> Gain/1
  Constant1/1 -> Sum6/1
  Trigonometric Function1/1 -> Sum6/2
  Sum6/1 -> Product/1
  Trigonometric Function2/1 -> Product/2
  MinMax/1 -> Product/3
  Input/1 -> Bus Selector3/1, Bus Selector4/1, Bus Selector1/1, Bus Selector2/1, Bus Selector5/1
  Gain/1 -> Sum1/3
  Sum1/1 -> MCV/1
  Bus Selector4/1 -> Sum1/2  "<Qb_rps>"
  Bus Selector1/1 -> Sum2/1  "<nz_g>"
  Constant2/1 -> Sum2/2
  Sum2/1 -> Product1/2
  Bus Selector2/1 -> Lookup Table/1, Lookup Table1/1, MinMax1/1  "<VT_mps>"
  Product1/1 -> Sum3/2
  Sum3/1 -> Sum1/1
  Lookup Table1/1 -> Product2/2
  Bus Selector5/1 -> Product2/1  "<ALPHA_rad>"
  Product2/1 -> Sum3/1
  Constant3/1 -> MinMax1/2
  Lookup Table/1 -> Product3/1
  MinMax1/1 -> Product3/2
  Product3/1 -> Gain2/1
  Gain2/1 -> Product1/1

== system admire_sim_NDI/NDI_CLAW/DynamicInversionControl/REG/PitchReg/GAMMACMD_2/GetGamma ==
  ANGLES : Inport
  Bus Selector1 : BusSelector  OutputSignals=ALPHA_rad,BETA_rad,THETA_rad
  Bus Selector2 : BusSelector  OutputSignals=PHI_rad,BETA_rad
  Bus Selector3 : BusSelector  OutputSignals=PHI_rad,ALPHA_rad,BETA_rad
  Bus Selector4 : BusSelector  OutputSignals=THETA_rad
  Product : Product  Inputs=3  RndMeth=Zero
  Product1 : Product  RndMeth=Zero
  Product2 : Product  Inputs=3  RndMeth=Zero
  Product3 : Product  RndMeth=Zero
  Sum : Sum  Inputs=|+-
  Sum1 : Sum  Inputs=|++
  Trigonometric Function{1,5..7,9} (5 alike) : Trigonometry  Operator=cos
  Trigonometric Function10 : Trigonometry  Operator=asin
  Trigonometric Function{2..4,8} (4 alike) : Trigonometry
  GAMMA_rad : Outport
  wires:
  Sum/1 -> Trigonometric Function10/1
  ANGLES/1 -> Bus Selector2/1, Bus Selector3/1, Bus Selector1/1, Bus Selector4/1
  Bus Selector1/1 -> Trigonometric Function9/1  "<ALPHA_rad>"
  Bus Selector1/2 -> Trigonometric Function1/1  "<BETA_rad>"
  Bus Selector1/3 -> Trigonometric Function8/1  "<THETA_rad>"
  Trigonometric Function9/1 -> Product/1
  Trigonometric Function1/1 -> Product/2
  Trigonometric Function8/1 -> Product/3
  Bus Selector2/1 -> Trigonometric Function2/1  "<PHI_rad>"
  Bus Selector2/2 -> Trigonometric Function3/1  "<BETA_rad>"
  Trigonometric Function2/1 -> Product1/1
  Trigonometric Function3/1 -> Product1/2
  Bus Selector3/2 -> Trigonometric Function4/1  "<ALPHA_rad>"
  Trigonometric Function6/1 -> Product2/1
  Trigonometric Function4/1 -> Product2/2
  Trigonometric Function5/1 -> Product2/3
  Bus Selector3/1 -> Trigonometric Function6/1  "<PHI_rad>"
  Bus Selector3/3 -> Trigonometric Function5/1  "<BETA_rad>"
  Product1/1 -> Sum1/1
  Product2/1 -> Sum1/2
  Bus Selector4/1 -> Trigonometric Function7/1  "<THETA_rad>"
  Sum1/1 -> Product3/2
  Product/1 -> Sum/1
  Product3/1 -> Sum/2
  Trigonometric Function7/1 -> Product3/1
  Trigonometric Function10/1 -> GAMMA_rad/1  "GAMMA_rad"

== system admire_sim_NDI/NDI_CLAW/DynamicInversionControl/REG/RollReg/PHIcmd_2/Get_LCV ==
  Input : Inport
  Bus Selector1 : BusSelector  OutputSignals=Pb_rps,ALPHA_rad,Rb_rps
  Product : Product  RndMeth=Zero
  Product1 : Product  RndMeth=Zero
  Sum3 : Sum  Inputs=|++
  Trigonometric Function : Trigonometry
  Trigonometric Function1 : Trigonometry  Operator=cos
  LCV : Outport
  wires:
  Bus Selector1/2 -> Trigonometric Function/1, Trigonometric Function1/1  "<ALPHA_rad>"
  Bus Selector1/1 -> Product/1  "<Pb_rps>"
  Trigonometric Function1/1 -> Product/2
  Trigonometric Function/1 -> Product1/1
  Bus Selector1/3 -> Product1/2  "<Rb_rps>"
  Product/1 -> Sum3/1
  Product1/1 -> Sum3/2
  Input/1 -> Bus Selector1/1
  Sum3/1 -> LCV/1

== system admire_sim_NDI/NDI_CLAW/DynamicInversionControl/REG/RollReg/PHIcmd_2/VariableLimiter ==
  Input : Inport
  Limit : Inport  Port=2
  Gain : Gain  Gain=-1
  MinMax : MinMax  Inputs=2
  MinMax1 : MinMax  Function=max  Inputs=2
  Out : Outport
  wires:
  MinMax/1 -> MinMax1/1
  Gain/1 -> MinMax1/2
  Input/1 -> MinMax/1
  Limit/1 -> MinMax/2, Gain/1
  MinMax1/1 -> Out/1

== system admire_sim_NDI/NDI_CLAW/DynamicInversionControl/REG/RollReg/Pcmd_1/Get_LCV ==
  Input : Inport
  Bus Selector1 : BusSelector  OutputSignals=Pb_rps,ALPHA_rad,Rb_rps
  Product : Product  RndMeth=Zero
  Product1 : Product  RndMeth=Zero
  Sum3 : Sum  Inputs=|++
  Trigonometric Function : Trigonometry
  Trigonometric Function1 : Trigonometry  Operator=cos
  LCV : Outport
  wires:
  Sum3/1 -> LCV/1
  Input/1 -> Bus Selector1/1
  Product1/1 -> Sum3/2
  Product/1 -> Sum3/1
  Bus Selector1/3 -> Product1/2  "<Rb_rps>"
  Trigonometric Function/1 -> Product1/1
  Trigonometric Function1/1 -> Product/2
  Bus Selector1/1 -> Product/1  "<Pb_rps>"
  Bus Selector1/2 -> Trigonometric Function1/1, Trigonometric Function/1  "<ALPHA_rad>"

== system admire_sim_NDI/NDI_CLAW/DynamicInversionControl/REG/RollReg/Pcmd_1/VariableLimiter ==
  Input : Inport
  Limit : Inport  Port=2
  Gain : Gain  Gain=-1
  MinMax : MinMax  Inputs=2
  MinMax1 : MinMax  Function=max  Inputs=2
  Out : Outport
  wires:
  MinMax1/1 -> Out/1
  Limit/1 -> Gain/1, MinMax/2
  Input/1 -> MinMax/1
  Gain/1 -> MinMax1/2
  MinMax/1 -> MinMax1/1

== system admire_sim_NDI/NDI_CLAW/DynamicInversionControl/REG/RollReg/XTKcmd_3/GetPHIcmd ==
  CMD : Inport
  INPUT : Inport  Port=2
  AcquireHeading : Subsystem
  Crosstrack : Subsystem
  Switch2 : Switch  Criteria=u2 > Threshold
  PHIcmd : Outport
  wires:
  CMD/1 -> AcquireHeading/2(CMD), Crosstrack/1(CMD)
  INPUT/1 -> AcquireHeading/1(INPUT), Crosstrack/2(INPUT)
  Switch2/1 -> PHIcmd/1
  Crosstrack/1(PHIcmd) -> Switch2/3
  AcquireHeading/1(PHIcmd_rad) -> Switch2/1
  AcquireHeading/2(Logic) -> Switch2/2

== system admire_sim_NDI/NDI_CLAW/DynamicInversionControl/REG/RollReg/XTKcmd_3/Get_LCV ==
  Input : Inport
  Bus Selector1 : BusSelector  OutputSignals=Pb_rps,ALPHA_rad,Rb_rps
  Product : Product  RndMeth=Zero
  Product1 : Product  RndMeth=Zero
  Sum3 : Sum  Inputs=|++
  Trigonometric Function : Trigonometry
  Trigonometric Function1 : Trigonometry  Operator=cos
  LCV : Outport
  wires:
  Sum3/1 -> LCV/1
  Input/1 -> Bus Selector1/1
  Product1/1 -> Sum3/2
  Product/1 -> Sum3/1
  Bus Selector1/3 -> Product1/2  "<Rb_rps>"
  Trigonometric Function/1 -> Product1/1
  Trigonometric Function1/1 -> Product/2
  Bus Selector1/1 -> Product/1  "<Pb_rps>"
  Bus Selector1/2 -> Trigonometric Function1/1, Trigonometric Function/1  "<ALPHA_rad>"

== system admire_sim_NDI/NDI_CLAW/DynamicInversionControl/REG/RollReg/XTKcmd_3/VariableLimiter ==
  Input : Inport
  Limit : Inport  Port=2
  Gain : Gain  Gain=-1
  MinMax : MinMax  Inputs=2
  MinMax1 : MinMax  Function=max  Inputs=2
  Out : Outport
  wires:
  MinMax1/1 -> Out/1
  Limit/1 -> Gain/1, MinMax/2
  Input/1 -> MinMax/1
  Gain/1 -> MinMax1/2
  MinMax/1 -> MinMax1/1

== system admire_sim_NDI/NDI_CLAW/MissionManager/WaypointNavigation/ChangeWptNumber/GetTurnDist/GetHalfAngle ==
  WNz : Inport
  Bus Creator : BusCreator  Inputs=2
  Bus Selector1 : BusSelector  OutputSignals=Xcmd,Ycmd  OutputAsBus=on
  Bus Selector3 : BusSelector  OutputSignals=Xcmdm1,Ycmdm1  OutputAsBus=on
  Bus Selector4 : BusSelector  OutputSignals=Xcmdp1,Ycmdp1  OutputAsBus=on
  Bus Selector5 : BusSelector  OutputSignals=Xcmd,Ycmd  OutputAsBus=on
  Bus Selector6 : BusSelector  OutputSignals=V1,V2
  Bus Selector7 : BusSelector  OutputSignals=V1,V2
  Constant2 : Constant  Value=1e-10
  Dot Product : DotProduct  InputSameDT=on  OutDataTypeStr=Inherit: Inherit via internal rule
  Dot Product1 : DotProduct  InputSameDT=on  OutDataTypeStr=Inherit: Inherit via internal rule
  Dot Product2 : DotProduct  InputSameDT=on  OutDataTypeStr=Inherit: Inherit via internal rule
  Gain3 : Gain  Gain=0.5
  MinMax : MinMax  Function=max  Inputs=2
  Product5 : Product  RndMeth=Zero
  Product6 : Product  Inputs=*/  RndMeth=Zero
  Saturation1 : Saturate  UpperLimit=.9848  LowerLimit=-.9848
  Signal Specification : SignalSpecification  Dimensions=2
  Sqrt1 : Sqrt  SaturateOnIntegerOverflow=on
  Sqrt2 : Sqrt  SaturateOnIntegerOverflow=on
  Sum2 : Sum  Inputs=|-+
  Sum3 : Sum  Inputs=|+-
  Trigonometric Function2 : Trigonometry  Operator=acos
  Out1 : Outport
  wires:
  WNz/1 -> Bus Selector1/1, Bus Selector3/1, Bus Selector4/1, Bus Selector5/1
  Bus Selector1/1 -> Sum2/1
  Bus Selector3/1 -> Sum2/2
  Bus Selector4/1 -> Sum3/1
  Bus Selector5/1 -> Sum3/2
  Sum2/1 -> Signal Specification/1  "V1"
  Sum3/1 -> Bus Creator/2  "V2"
  Bus Creator/1 -> Bus Selector6/1, Bus Selector7/1
  Bus Selector6/1 -> Dot Product/1  "<V1>"
  Bus Selector6/2 -> Dot Product/2  "<V2>"
  Dot Product1/1 -> Sqrt1/1
  Dot Product2/1 -> Sqrt2/1
  Bus Selector7/1 -> Dot Product1/2, Dot Product1/1  "<V1>"
  Bus Selector7/2 -> Dot Product2/1, Dot Product2/2  "<V2>"
  Sqrt1/1 -> Product5/1
  Sqrt2/1 -> Product5/2
  Product5/1 -> MinMax/1
  Constant2/1 -> MinMax/2
  Dot Product/1 -> Product6/1
  MinMax/1 -> Product6/2
  Product6/1 -> Saturation1/1
  Saturation1/1 -> Trigonometric Function2/1
  Trigonometric Function2/1 -> Gain3/1
  Gain3/1 -> Out1/1
  Signal Specification/1 -> Bus Creator/1

== system admire_sim_NDI/NDI_CLAW/MissionManager/WaypointNavigation/ChangeWptNumber/GetTurnDist/GetPHILimit ==
  note: Load factor at CLmax
  note: Limit to 9 g's for structure
  note: Only use 80% to leave
      | margin to avoid stall
      |
      | Change to 100% to investigate
      | maximum performance turns
  V2 : Inport
  Gain : Gain  Gain=0.5*Sref*1.5*.65/(mass*9.81)
  Gain3 : Gain  Gain=0.8
  Product1 : Product  Inputs=/  RndMeth=Zero
  Saturation : Saturate  UpperLimit=9  LowerLimit=1.015
  Trigonometric Function : Trigonometry  Operator=acos
  PHImax_rad : Outport
  wires:
  Gain/1 -> Saturation/1  "n"
  Saturation/1 -> Product1/1
  Product1/1 -> Trigonometric Function/1
  Trigonometric Function/1 -> Gain3/1
  V2/1 -> Gain/1
  Gain3/1 -> PHImax_rad/1  "PHImax_rad"

== system admire_sim_NDI/NDI_CLAW/MissionManager/WaypointNavigation/ChangeWptNumber/GetTurnDist/GetRadius ==
  V2 : Inport
  PHImax_rad : Inport  Port=2
  Constant1 : Constant
  Gain2 : Gain  Gain=9.81
  Product2 : Product  Inputs=/  RndMeth=Zero
  Product3 : Product  RndMeth=Zero
  Product4 : Product  Inputs=*/  RndMeth=Zero
  Sqrt : Sqrt  SaturateOnIntegerOverflow=on
  Sum1 : Sum  Inputs=|+-
  Trigonometric Function1 : Trigonometry  Operator=cos
  R_m : Outport
  wires:
  Trigonometric Function1/1 -> Product2/1
  Product2/1 -> Product3/1, Product3/2
  Product3/1 -> Sum1/1
  Constant1/1 -> Sum1/2
  Sum1/1 -> Sqrt/1
  Sqrt/1 -> Gain2/1
  Gain2/1 -> Product4/2
  Product4/1 -> R_m/1  "R_m"
  V2/1 -> Product4/1
  PHImax_rad/1 -> Trigonometric Function1/1

== system admire_sim_NDI/NDI_CLAW/DynamicInversionControl/AERO_OBM/NonLinearOBM/Get_B_Aero/Dimensions/GetDensity ==
  Alt_m : Inport
  Constant : Constant  Value=288.15
  Constant1 : Constant  Value=5.2561
  Constant2 : Constant
  Gain : Gain  Gain=0.0065
  Gain1 : Gain  Gain=0.0065/288.15
  Gain2 : Gain  Gain=101325
  Gain9 : Gain  Gain=287.04
  Math Function : Math  Operator=pow  SaturateOnIntegerOverflow=on
  Product2 : Product  Inputs=*/  RndMeth=Zero
  Sum : Sum  Inputs=|+-
  Sum2 : Sum  Inputs=|+-
  rho_kpm3 : Outport
  wires:
  Constant/1 -> Sum/1
  Gain/1 -> Sum/2
  Alt_m/1 -> Gain1/1, Gain/1
  Constant2/1 -> Sum2/1
  Gain1/1 -> Sum2/2
  Sum2/1 -> Math Function/1
  Constant1/1 -> Math Function/2
  Math Function/1 -> Gain2/1
  Sum/1 -> Gain9/1  "T_K"
  Gain2/1 -> Product2/1  "P_npm2"
  Gain9/1 -> Product2/2
  Product2/1 -> rho_kpm3/1

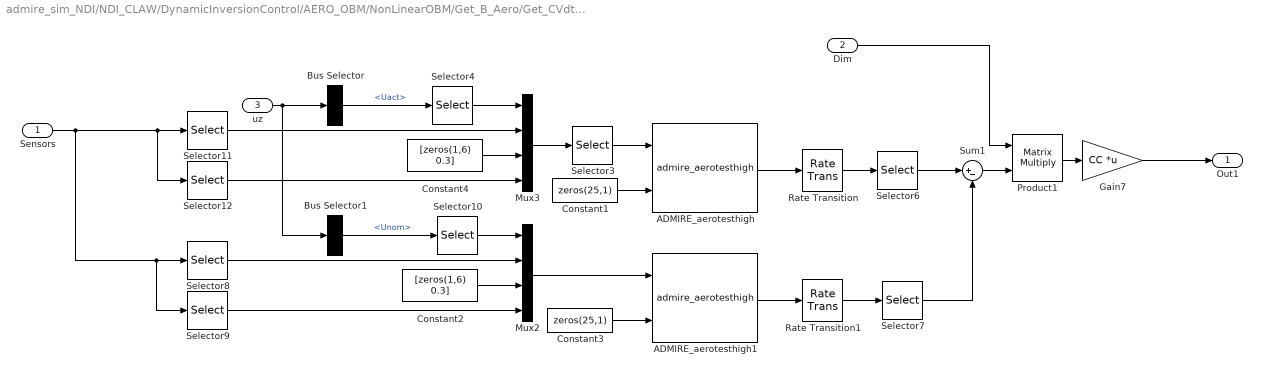
== system admire_sim_NDI/NDI_CLAW/DynamicInversionControl/AERO_OBM/NonLinearOBM/Get_B_Aero/Get_CVdt/DueToEffectors ==
  Sensors : Inport
  Dim : Inport  Port=2
  uz : Inport  Port=3
  ADMIRE_aerotesthigh : S-Function  FunctionName=admire_aerotesthigh  SFunctionDeploymentMode=off  EnableBusSupport=off
  ADMIRE_aerotesthigh1 : S-Function  FunctionName=admire_aerotesthigh  SFunctionDeploymentMode=off  EnableBusSupport=off
  Bus Selector : BusSelector  OutputSignals=Uact
  Bus Selector1 : BusSelector  OutputSignals=Unom
  Constant1 : Constant  Value=zeros(25,1)
  Constant2 : Constant  Value=[zeros(1,6) 0.3]
  Constant3 : Constant  Value=zeros(25,1)
  Constant4 : Constant  Value=[zeros(1,6) 0.3]
  Gain7 : Gain  Gain=CC  Multiplication=Matrix(K*u)
  Mux2 : Mux
  Mux3 : Mux
  Product1 : Product  Multiplication=Matrix(*)
  Rate Transition : RateTransition  OutPortSampleTime=dt
  Rate Transition1 : RateTransition  OutPortSampleTime=dt
  Selector10 : Selector  InputPortWidth=16  IndexOptions=Index vector (dialog)  Indices=[1:8 10 9 11 12]  OutputSizes=1
  Selector11 : Selector  InputPortWidth=28  IndexOptions=Index vector (dialog)  Indices=[1:6 12]  OutputSizes=1
  Selector12 : Selector  InputPortWidth=28  IndexOptions=Index vector (dialog)  Indices=[19]  OutputSizes=1
  Selector3 : Selector  NumberOfDimensions=2  InputPortWidth=3  IndexOptions=Index vector (dialog),Index vector (dialog)  Indices=[1:27],1  OutputSizes=1,1
  Selector4 : Selector  InputPortWidth=16  IndexOptions=Index vector (dialog)  Indices=[1:8 10 9 11 12]  OutputSizes=1
  Selector6 : Selector  InputPortWidth=9  IndexOptions=Index vector (dialog)  Indices=[4:6]  OutputSizes=1
  Selector7 : Selector  InputPortWidth=9  IndexOptions=Index vector (dialog)  Indices=[4:6]  OutputSizes=1
  Selector8 : Selector  InputPortWidth=28  IndexOptions=Index vector (dialog)  Indices=[1:6 12]  OutputSizes=1
  Selector9 : Selector  InputPortWidth=28  IndexOptions=Index vector (dialog)  Indices=[19]  OutputSizes=1
  Sum1 : Sum  Inputs=|+-
  Out1 : Outport
  wires:
  Mux2/1 -> ADMIRE_aerotesthigh1/1
  ADMIRE_aerotesthigh/1 -> Rate Transition/1
  Constant1/1 -> ADMIRE_aerotesthigh/2
  Constant3/1 -> ADMIRE_aerotesthigh1/2
  Selector3/1 -> ADMIRE_aerotesthigh/1
  uz/1 -> Bus Selector/1, Bus Selector1/1
  Product1/1 -> Gain7/1
  Dim/1 -> Product1/1
  Sum1/1 -> Product1/2
  Mux3/1 -> Selector3/1
  Selector12/1 -> Mux3/4
  Selector4/1 -> Mux3/1
  Constant4/1 -> Mux3/3
  Selector11/1 -> Mux3/2
  ADMIRE_aerotesthigh1/1 -> Rate Transition1/1
  Selector6/1 -> Sum1/1
  Selector9/1 -> Mux2/4
  Selector8/1 -> Mux2/2
  Sensors/1 -> Selector9/1, Selector8/1, Selector11/1, Selector12/1
  Constant2/1 -> Mux2/3
  Selector10/1 -> Mux2/1
  Gain7/1 -> Out1/1
  Selector7/1 -> Sum1/2
  Rate Transition/1 -> Selector6/1
  Rate Transition1/1 -> Selector7/1
  Bus Selector/1 -> Selector4/1  "<Uact>"
  Bus Selector1/1 -> Selector10/1  "<Unom>"

== system admire_sim_NDI/NDI_CLAW/DynamicInversionControl/AERO_OBM/NonLinearOBM/Get_B_Aero/Get_CVdt/TotalAccels ==
  Dim : Inport
  Sensors : Inport  Port=2
  Bus Creator2 : BusCreator  Inputs=6
  Bus Creator3 : BusCreator  Inputs=3
  Demux1 : Demux  Outputs=3
  Demux4 : Demux  Outputs=3
  Get_Pbdt1 : Subsystem
  Get_Qbdt1 : Subsystem
  Get_Rbdt1 : Subsystem
  Product2 : Product  Multiplication=Matrix(*)  RndMeth=Zero
  Selector4 : Selector  InputPortWidth=28  IndexOptions=Index vector (dialog)  Indices=[4:6]  OutputSizes=1
  Selector5 : Selector  InputPortWidth=28  IndexOptions=Index vector (dialog)  Indices=[26:28]  OutputSizes=1
  CVdt : Outport
  wires:
  Demux1/1 -> Bus Creator2/1  "Pb"
  Demux1/2 -> Bus Creator2/2  "Qb"
  Demux1/3 -> Bus Creator2/3  "Rb"
  Demux4/1 -> Bus Creator2/4  "Mx"
  Demux4/3 -> Bus Creator2/6  "Mz"
  Selector4/1 -> Demux1/1
  Selector5/1 -> Product2/2
  Dim/1 -> Product2/1
  Get_Pbdt1/1(Pbdt) -> Bus Creator3/1
  Get_Qbdt1/1(Qbdt) -> Bus Creator3/2
  Get_Rbdt1/1(Rbdt) -> Bus Creator3/3
  Bus Creator2/1 -> Get_Pbdt1/1(In1), Get_Qbdt1/1(In1), Get_Rbdt1/1(In1)
  Sensors/1 -> Selector4/1, Selector5/1
  Bus Creator3/1 -> CVdt/1
  Product2/1 -> Demux4/1
  Demux4/2 -> Bus Creator2/5  "My"

== system admire_sim_NDI/NDI_CLAW/DynamicInversionControl/AERO_OBM/NonLinearOBM/Get_B_Aero/OneColPerFrame/u1 ==
  In1 : Inport
  Action Port : ActionPort  ActionType=case
  ADMIRE_aerotesthigh : S-Function  FunctionName=admire_aerotesthigh  SFunctionDeploymentMode=off  EnableBusSupport=off
  ADMIRE_aerotesthigh1 : S-Function  FunctionName=admire_aerotesthigh  SFunctionDeploymentMode=off  EnableBusSupport=off
  Constant1 : Constant  Value=zeros(25,1)
  Gain : Gain  Gain=0.5*r2d
  Selector : Selector  NumberOfDimensions=2  InputPortWidth=3  IndexOptions=Index vector (dialog),Index vector (dialog)  Indices=[1:27],1  OutputSizes=1,1
  Selector1 : Selector  NumberOfDimensions=2  InputPortWidth=3  IndexOptions=Index vector (dialog),Index vector (dialog)  Indices=[1:27],8  OutputSizes=1,1
  Selector2 : Selector  InputPortWidth=9  IndexOptions=Index vector (dialog)  Indices=[4:6]  OutputSizes=1
  Selector3 : Selector  InputPortWidth=9  IndexOptions=Index vector (dialog)  Indices=[4:6]  OutputSizes=1
  Sum1 : Sum  Inputs=|+-
  Out1 : Outport
  wires:
  Gain/1 -> Out1/1
  Selector3/1 -> Sum1/2
  Selector2/1 -> Sum1/1
  Sum1/1 -> Gain/1
  ADMIRE_aerotesthigh1/1 -> Selector3/1
  ADMIRE_aerotesthigh/1 -> Selector2/1
  Selector1/1 -> ADMIRE_aerotesthigh1/1
  Selector/1 -> ADMIRE_aerotesthigh/1
  In1/1 -> Selector/1, Selector1/1
  Constant1/1 -> ADMIRE_aerotesthigh/2, ADMIRE_aerotesthigh1/2

== system admire_sim_NDI/NDI_CLAW/DynamicInversionControl/AERO_OBM/NonLinearOBM/Get_B_Aero/OneColPerFrame/u2 ==
  In1 : Inport
  Action Port : ActionPort  ActionType=case
  ADMIRE_aerotesthigh : S-Function  FunctionName=admire_aerotesthigh  SFunctionDeploymentMode=off  EnableBusSupport=off
  ADMIRE_aerotesthigh1 : S-Function  FunctionName=admire_aerotesthigh  SFunctionDeploymentMode=off  EnableBusSupport=off
  Constant1 : Constant  Value=zeros(25,1)
  Gain : Gain  Gain=0.5*r2d
  Selector : Selector  NumberOfDimensions=2  InputPortWidth=3  IndexOptions=Index vector (dialog),Index vector (dialog)  Indices=[1:27],2  OutputSizes=1,1
  Selector1 : Selector  NumberOfDimensions=2  InputPortWidth=3  IndexOptions=Index vector (dialog),Index vector (dialog)  Indices=[1:27],9  OutputSizes=1,1
  Selector2 : Selector  InputPortWidth=9  IndexOptions=Index vector (dialog)  Indices=[4:6]  OutputSizes=1
  Selector3 : Selector  InputPortWidth=9  IndexOptions=Index vector (dialog)  Indices=[4:6]  OutputSizes=1
  Sum1 : Sum  Inputs=|+-
  Out1 : Outport
  wires:
  Constant1/1 -> ADMIRE_aerotesthigh/2, ADMIRE_aerotesthigh1/2
  In1/1 -> Selector1/1, Selector/1
  Selector/1 -> ADMIRE_aerotesthigh/1
  Selector1/1 -> ADMIRE_aerotesthigh1/1
  ADMIRE_aerotesthigh/1 -> Selector2/1
  ADMIRE_aerotesthigh1/1 -> Selector3/1
  Sum1/1 -> Gain/1
  Selector2/1 -> Sum1/1
  Selector3/1 -> Sum1/2
  Gain/1 -> Out1/1

== system admire_sim_NDI/NDI_CLAW/DynamicInversionControl/AERO_OBM/NonLinearOBM/Get_B_Aero/OneColPerFrame/u3 ==
  In1 : Inport
  Action Port : ActionPort  ActionType=case
  ADMIRE_aerotesthigh : S-Function  FunctionName=admire_aerotesthigh  SFunctionDeploymentMode=off  EnableBusSupport=off
  ADMIRE_aerotesthigh1 : S-Function  FunctionName=admire_aerotesthigh  SFunctionDeploymentMode=off  EnableBusSupport=off
  Constant1 : Constant  Value=zeros(25,1)
  Gain : Gain  Gain=0.5*r2d
  Selector : Selector  NumberOfDimensions=2  InputPortWidth=3  IndexOptions=Index vector (dialog),Index vector (dialog)  Indices=[1:27],3  OutputSizes=1,1
  Selector1 : Selector  NumberOfDimensions=2  InputPortWidth=3  IndexOptions=Index vector (dialog),Index vector (dialog)  Indices=[1:27],10  OutputSizes=1,1
  Selector2 : Selector  InputPortWidth=9  IndexOptions=Index vector (dialog)  Indices=[4:6]  OutputSizes=1
  Selector3 : Selector  InputPortWidth=9  IndexOptions=Index vector (dialog)  Indices=[4:6]  OutputSizes=1
  Sum1 : Sum  Inputs=|+-
  Out1 : Outport
  wires:
  Gain/1 -> Out1/1
  Selector3/1 -> Sum1/2
  Selector2/1 -> Sum1/1
  Sum1/1 -> Gain/1
  ADMIRE_aerotesthigh1/1 -> Selector3/1
  ADMIRE_aerotesthigh/1 -> Selector2/1
  Selector1/1 -> ADMIRE_aerotesthigh1/1
  Selector/1 -> ADMIRE_aerotesthigh/1
  In1/1 -> Selector/1, Selector1/1
  Constant1/1 -> ADMIRE_aerotesthigh/2, ADMIRE_aerotesthigh1/2
